simulink model "quadsim"  (R2023a)
settings: Solver=FixedStepAuto  StartTime=0.0  StopTime=tf  FixedStep=tstep  RelTol=1e-3  EnableMultiTasking=on
values from neighbouring files (symbols this model uses):
  con = [m,g,Ixx,Iyy,Izz,Ixy,Ixz,Iyz]    [main.m]
  con_real = [m_real,g_real,Ixx_real,Iyy_real,Izz_real,Ixy_real,Ixz_real,Iyz_real]    [main.m]
  KA = [-22.3606698191395	0.00201472423721912	-0.0210042926161882	-5.14256360667609	-0.00544994639254871	-0.00539750017780217	-0.591349567789534	2.56742275495149e-08	-0.000222035484653320 ... (first row only)    [main.m]
  KT = [0.0719636752505308	-0.0719636752505340	3.14585832307952	0.205167084974015	-0.205167084974022	5.80096376452051	-0.215718994756261	0.215718994756262	5.40168970403702 ... (first row only)    [main.m]
  l = 0.2    [Attitude.m]
  LA = [4.47090494564492	1.24715387948497e-08	0.00499221978617721	0.744440755445128	-4.66935645274561e-05	0.00155055930580347; 1.24715387948497e-08	4.47089657692810	5.57847618618385e-06	4.66676478608033e-05	0.744439338778690	1.57839222690215e-05; 0.00499221978617721	5.57847618618385e-06	4.46797672976086	0.000844876774321680	-2.51353961198021e-05	1.36306650125613; 0.0148888151089026	9.33352957216066e-07	1 ...(+321 chars)    [main.m]
  LT = [31.6173277650076	8.77856768873147e-05	-0.000368035074502750	1.84128362143915	3.68731318527742e-06	0.235633602584559; 8.77856768873147e-05	31.6173277650076	0.000368035074499152	3.68731318640445e-06	1.84128362143917	-0.235633602584566; -0.000368035074502750	0.000368035074499152	31.6135634683629	-0.180767234820393	0.180767234820397	2.40014416703265; 0.184128362143915	3.68731318640445e-07	-0.01807672 ...(+309 chars)    [main.m]
  ref = [pi/18 pi/32 0]    [Attitude.m]    (also in Translational.m = [0 0 -2]; main.m = [1;1;-2])
  tstep = 0.001    [ActuatorModel.m]    (also in Attitude.m; Translational.m; UpdatedAttitude.m = 0.0001; main.m)
  x0 = [0; 0; 0]    [UpdatedAttitude.m]    (also in main.m = [0;0;0;0;0;0;0;0;0;0;0;0])
undefined symbols (not defined in the file or in its folder): k1, k2, wmax
libraries: simulink x1
settings Model: Creator=Nathan Dablain  LastModifiedBy=Nathan Dablain

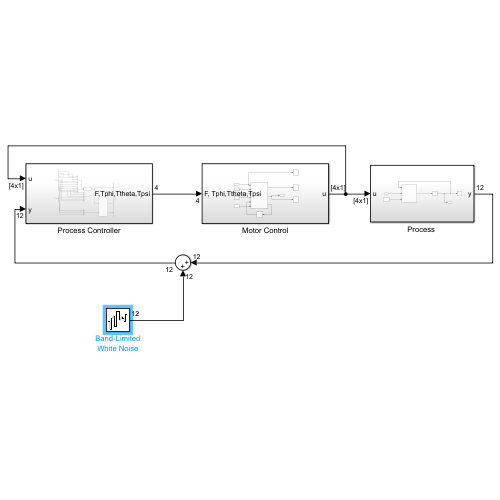
[thumbnail: Simulink's stored preview of the top-level diagram]
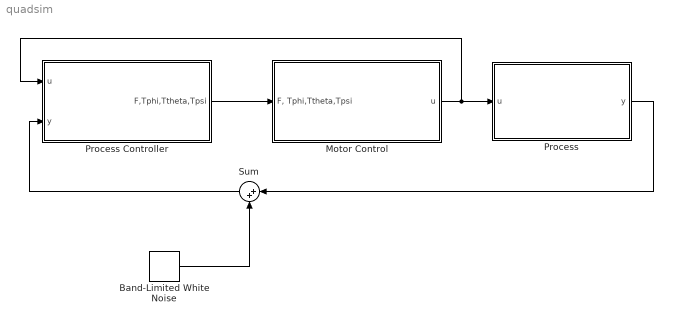
== system quadsim ==
  Band-Limited White Noise : simulink/Sources/Band-Limited White Noise  Cov=[1e-4 1e-4 1e-4 5e-5 5e-6 5e-6 1e-5 1e-5 1e-5 1e-6 1e-6 1e-6]  Ts=tstep  seed=[23341]
  Motor Control : Subsystem
  "Process " : Subsystem
  Process Controller : Subsystem
  Sum : Sum  Inputs=|++
  wires:
  Process Controller/1(F,Tphi,Ttheta,Tpsi) -> Motor Control/1("F, Tphi,Ttheta,Tpsi")
  Motor Control/1(u) -> Process Controller/1(u), "Process "/1(u)
  "Process "/1(y) -> Sum/1
  Band-Limited White Noise/1 -> Sum/2
  Sum/1 -> Process Controller/2(y)

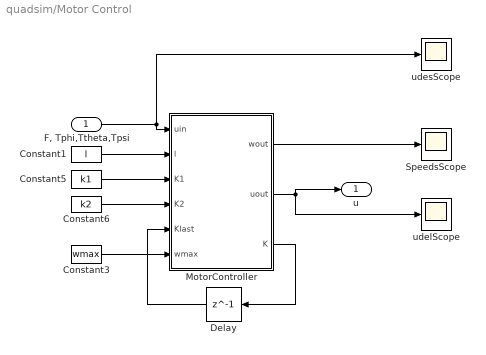
== system quadsim/Motor Control ==
  "F, Tphi,Ttheta,Tpsi" : Inport
  Constant1 : Constant  Value=l
  Constant3 : Constant  Value=wmax
  Constant5 : Constant  Value=k1
  Constant6 : Constant  Value=k2
  Delay : Delay  DelayLength=1  InitialCondition=1e-6.*ones(1,8)
  MotorController : MATLAB Function  TreatAsAtomicUnit=on
  SpeedsScope : Scope
  udelScope : Scope
  udesScope : Scope
  u : Outport
  wires:
  Constant1/1 -> MotorController/2(l)
  "F, Tphi,Ttheta,Tpsi"/1 -> udesScope/1, MotorController/1(uin)
  MotorController/2(uout) -> udelScope/1, u/1
  Constant3/1 -> MotorController/6(wmax)
  Constant5/1 -> MotorController/3(K1)
  Constant6/1 -> MotorController/4(K2)
  MotorController/1(wout) -> SpeedsScope/1
  MotorController/3(K) -> Delay/1
  Delay/1 -> MotorController/5(Klast)

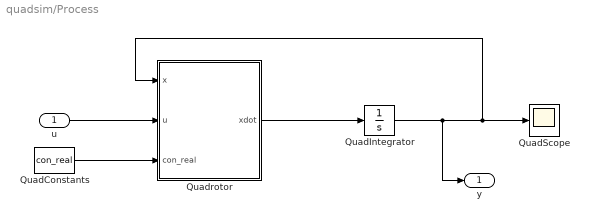
== system quadsim/Process  ==
  u : Inport
  QuadConstants : Constant  Value=con_real
  QuadIntegrator : Integrator  InitialCondition=x0
  QuadScope : Scope
  Quadrotor : MATLAB Function  TreatAsAtomicUnit=on
  y : Outport
  wires:
  u/1 -> Quadrotor/2(u)
  Quadrotor/1(xdot) -> QuadIntegrator/1
  QuadConstants/1 -> Quadrotor/3(con_real)
  QuadIntegrator/1 -> y/1, QuadScope/1, Quadrotor/1(x)

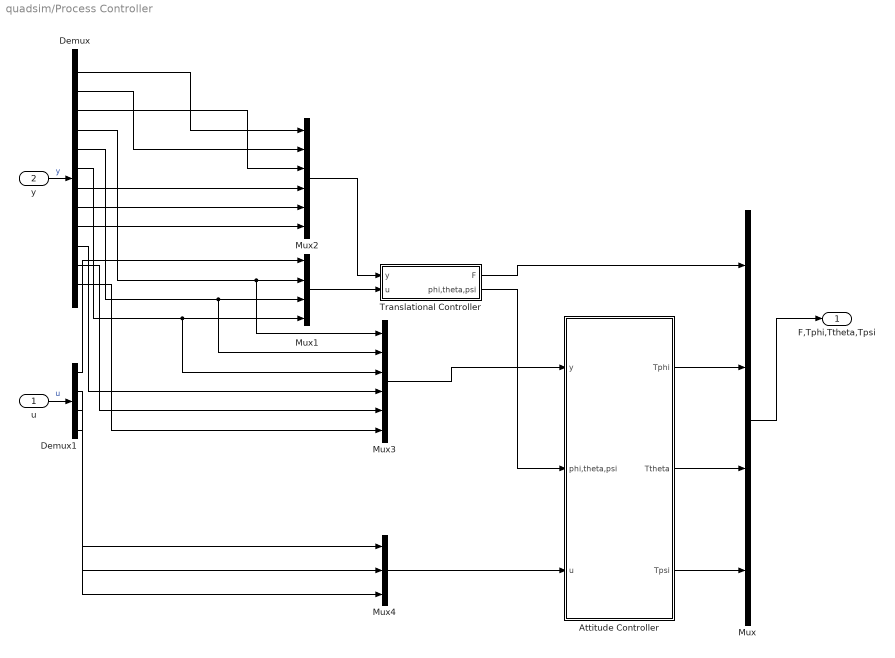
== system quadsim/Process Controller ==
  u : Inport
  y : Inport  Port=2
  Attitude Controller : Subsystem
  Demux : Demux  Outputs=12
  Demux1 : Demux
  Mux : Mux
  Mux1 : Mux
  Mux2 : Mux  Inputs=6
  Mux3 : Mux  Inputs=6
  Mux4 : Mux  Inputs=3
  Translational Controller : Subsystem
  F,Tphi,Ttheta,Tpsi : Outport
  wires:
  Mux/1 -> F,Tphi,Ttheta,Tpsi/1
  Translational Controller/1(F) -> Mux/1
  Attitude Controller/1(Tphi) -> Mux/2
  Attitude Controller/2(Ttheta) -> Mux/3
  Attitude Controller/3(Tpsi) -> Mux/4
  Translational Controller/2(phi,theta,psi) -> Attitude Controller/2(phi,theta,psi)
  Mux1/1 -> Translational Controller/2(u)
  Mux2/1 -> Translational Controller/1(y)
  Mux3/1 -> Attitude Controller/1(y)
  y/1 -> Demux/1  "y"
  u/1 -> Demux1/1  "u"
  Demux/1 -> Mux2/1
  Demux/2 -> Mux2/2
  Demux/3 -> Mux2/3
  Demux/7 -> Mux2/4
  Demux/8 -> Mux2/5
  Demux/9 -> Mux2/6
  Demux1/1 -> Mux1/1
  Demux/4 -> Mux3/1, Mux1/2
  Demux/5 -> Mux3/2, Mux1/3
  Demux/6 -> Mux3/3, Mux1/4
  Mux4/1 -> Attitude Controller/3(u)
  Demux1/2 -> Mux4/1
  Demux1/3 -> Mux4/2
  Demux1/4 -> Mux4/3
  Demux/10 -> Mux3/4
  Demux/11 -> Mux3/5
  Demux/12 -> Mux3/6

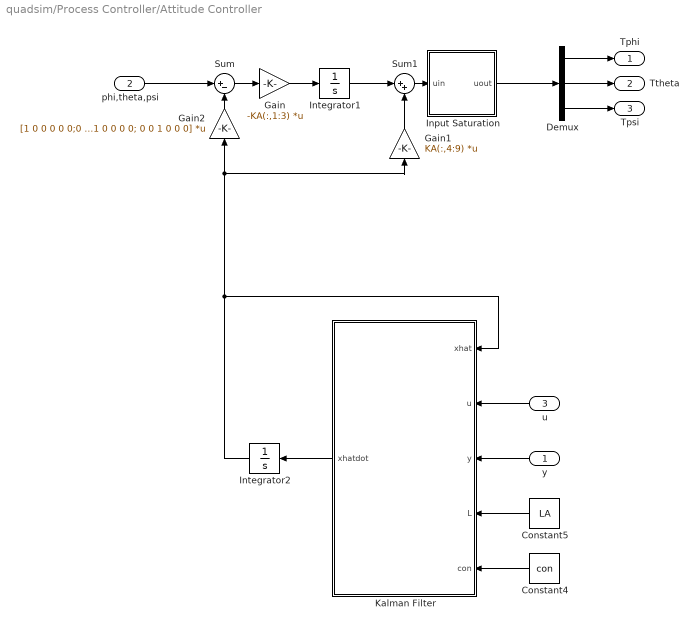
== system quadsim/Process Controller/Attitude Controller ==
  y : Inport
  phi,theta,psi : Inport  Port=2
  u : Inport  Port=3
  Constant4 : Constant  Value=con
  Constant5 : Constant  Value=LA
  Demux : Demux  Outputs=3
  Gain : Gain  Gain=-KA(:,1:3)  Multiplication=Matrix(K*u)
  Gain1 : Gain  Gain=KA(:,4:9)  Multiplication=Matrix(K*u)
  Gain2 : Gain  Gain=[1 0 0 0 0 0;0 1 0 0 0 0; 0 0 1 0 0 0]  Multiplication=Matrix(K*u)
  Input Saturation : MATLAB Function  TreatAsAtomicUnit=on
  Integrator1 : Integrator  InitialCondition=zeros(3,1)
  Integrator2 : Integrator  InitialCondition=zeros(6,1)
  Kalman Filter : MATLAB Function  TreatAsAtomicUnit=on
  Sum : Sum  Inputs=|+-
  Sum1 : Sum  Inputs=|++
  Tphi : Outport
  Ttheta : Outport  Port=2
  Tpsi : Outport  Port=3
  wires:
  phi,theta,psi/1 -> Sum/1
  Sum/1 -> Gain/1
  Gain/1 -> Integrator1/1
  Input Saturation/1(uout) -> Demux/1
  Gain1/1 -> Sum1/2
  Sum1/1 -> Input Saturation/1(uin)
  Integrator1/1 -> Sum1/1
  Demux/1 -> Tphi/1
  Demux/2 -> Ttheta/1
  Demux/3 -> Tpsi/1
  Gain2/1 -> Sum/2
  Integrator2/1 -> Kalman Filter/1(xhat), Gain1/1, Gain2/1
  Constant4/1 -> Kalman Filter/5(con)
  Kalman Filter/1(xhatdot) -> Integrator2/1
  y/1 -> Kalman Filter/3(y)
  Constant5/1 -> Kalman Filter/4(L)
  u/1 -> Kalman Filter/2(u)

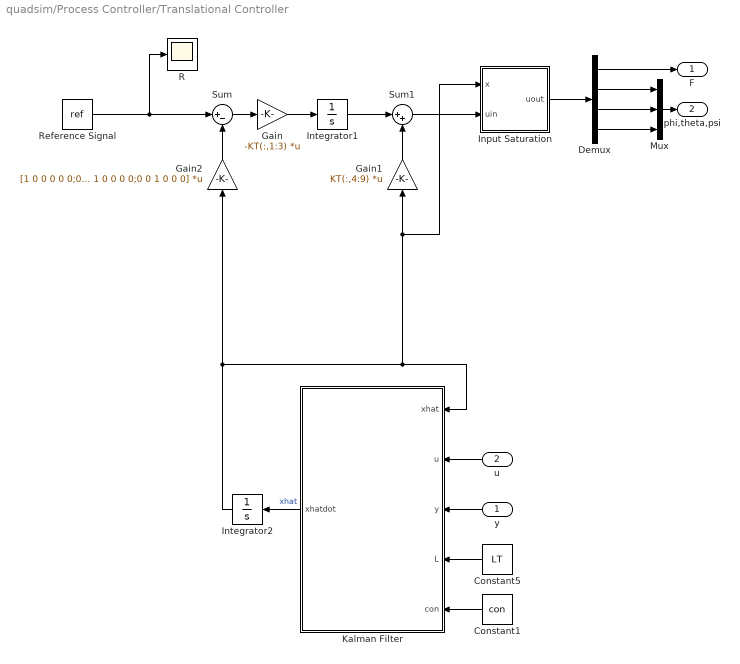
== system quadsim/Process Controller/Translational Controller ==
  y : Inport
  u : Inport  Port=2
  Constant1 : Constant  Value=con
  Constant5 : Constant  Value=LT
  Demux : Demux
  Gain : Gain  Gain=-KT(:,1:3)  Multiplication=Matrix(K*u)
  Gain1 : Gain  Gain=KT(:,4:9)  Multiplication=Matrix(K*u)
  Gain2 : Gain  Gain=[1 0 0 0 0 0;0 1 0 0 0 0;0 0 1 0 0 0]  Multiplication=Matrix(K*u)
  Input Saturation : MATLAB Function  TreatAsAtomicUnit=on
  Integrator1 : Integrator  InitialCondition=zeros(4,1)
  Integrator2 : Integrator  InitialCondition=zeros(6,1)
  Kalman Filter : MATLAB Function  TreatAsAtomicUnit=on
  Mux : Mux  Inputs=3
  R : Scope
  Reference Signal : Constant  Value=ref
  Sum : Sum  Inputs=|+-
  Sum1 : Sum  Inputs=|++
  F : Outport
  phi,theta,psi : Outport  Port=2
  wires:
  Sum1/1 -> Input Saturation/2(uin)
  Gain/1 -> Integrator1/1
  Sum/1 -> Gain/1
  Integrator1/1 -> Sum1/1
  Reference Signal/1 -> R/1, Sum/1
  Gain1/1 -> Sum1/2
  Input Saturation/1(uout) -> Demux/1
  Demux/1 -> F/1
  Demux/2 -> Mux/1
  Demux/3 -> Mux/2
  Demux/4 -> Mux/3
  Mux/1 -> phi,theta,psi/1
  Gain2/1 -> Sum/2
  Integrator2/1 -> Gain2/1, Input Saturation/1(x), Gain1/1, Kalman Filter/1(xhat)
  u/1 -> Kalman Filter/2(u)
  y/1 -> Kalman Filter/3(y)
  Constant5/1 -> Kalman Filter/4(L)
  Kalman Filter/1(xhatdot) -> Integrator2/1  "xhat"
  Constant1/1 -> Kalman Filter/5(con)

== matlab function quadsim/Process Controller/Translational Controller/Input Saturation ==
  data: x input; uin input; uout output
function uout = fcn(x,uin)
uout = uin;
max_ang = 20*pi/180; % rad
max_thrust = 30; % N
if uin(1)> max_thrust
    uout(1) = max_thrust;
elseif uin(1)<0
    uout(1) = 0;
end
for i = 2:4
    if x(3)>=-0.01
        uout(i) = 0;
    elseif uin(i) > max_ang
        uout(i) = max_ang;
    elseif uin(i) < -max_ang
        uout(i) = -max_ang;
    end
end
end

== matlab function quadsim/Process Controller/Attitude Controller/Kalman Filter ==
  data: xhat input; xhatdot output; u input; y input; L input; con input
function xhatdot  = fcn(xhat,u,y,L,con)
I = diag([con(3) con(4) con(5)]);
yhat = eye(6)*xhat;
xhatdot = [[1 sin(xhat(1))*tan(xhat(2)) cos(xhat(1))*tan(xhat(2));...
    0 cos(xhat(1)) -sin(xhat(1));...
    0 sin(xhat(1))*sec(xhat(2)) cos(xhat(1))*sec(xhat(2))]*xhat(4:6);...
    I\(u - cross(xhat(4:6),I*xhat(4:6)))] + L*(y-yhat);
end

== matlab function quadsim/Process Controller/Attitude Controller/Input Saturation ==
  data: uin input; uout output
function uout = fcn(uin)
uout = uin;
max_thrust = 30; % N
max_torque = max_thrust*0.2; % N-m
for i = 1:3
    if uin(i) > max_torque
        uout(i) = max_torque;
    elseif uin(i) < -max_torque
        uout(i) = -max_torque;
    end
end
end

== matlab function quadsim/Process Controller/Translational Controller/Kalman Filter ==
  data: xhat input; u input; y input; xhatdot output; L input; con input
function xhatdot   = fcn(xhat,u,y,L,con)
m = con(1);
g = con(2);

K = 5000; % Ground stiffness (N/m)
c = 150; % Ground damping (N/m/s)
if xhat(3) >= 0
    Fr = [c*xhat(4);c*xhat(5);K*xhat(3) + c*xhat(6)]; % Ground reaction force
else
    Fr = zeros(3,1);
end

phi = u(2);
theta = u(3);
psi = u(4);
yhat = eye(6)*xhat;
xhatdot = [[cos(theta)*cos(psi)  sin(phi)*sin(theta)*cos(psi) - cos(phi)*sin(psi) cos(phi)*sin(theta)*cos(psi)+sin(phi)*sin(psi);... 
    cos(theta)*sin(psi)  sin(phi)*sin(theta)*sin(psi)+cos(phi)*cos(psi) cos(phi)*sin(theta)*sin(psi)-sin(phi)*cos(psi);... 
    -sin(theta) sin(phi)*cos(theta) cos(phi)*cos(theta)]*xhat(4:6);...
    -g*sin(theta) - Fr(1)/m;...
    g*cos(theta)*sin(phi) - Fr(2)/m;...
    -u(1)/m-Fr(3)/m+g*cos(theta)*cos(phi)] + L*(y-yhat);
end

== matlab function quadsim/Motor Control/MotorController ==
  data: uin input; wout output; l input; K1 input; K2 input; Klast input; wmax input; uout output; K output
function [wout,uout, K] = fcn(uin, l, K1, K2, Klast, wmax)
w = zeros(4,1);
const = [Klast(1) Klast(2) Klast(3) Klast(4);...
    0 -l*Klast(2) 0 l*Klast(4);...
    -l*Klast(1) 0 l*Klast(3) 0;...
    -Klast(5) Klast(6) -Klast(7) Klast(8)];
w = const\uin;
for i = 1:4
    if w(i) <= 1
        w(i) = (2/60)^2;
    elseif sqrt(w(i))*60 >= wmax
        w(i) = (wmax/60)^2;
    end
end
K11 = K1(round(sqrt(w(1))*60)); %Because K is indexed based off of 0-7000 rpm, but n is in rps, w is rps^2
K12 = K1(round(sqrt(w(2))*60));
K13 = K1(round(sqrt(w(3))*60));
K14 = K1(round(sqrt(w(4))*60));
K21 = K2(round(sqrt(w(1))*60));
K22 = K2(round(sqrt(w(2))*60));
K23 = K2(round(sqrt(w(3))*60));
K24 = K2(round(sqrt(w(4))*60));
uout = [K11 K12 K13 K14;...
    0 -l*K12 0 l*K14;...
    -l*K11 0 l*K13 0;...
    -K21 K22 -K23 K24]*w;
wout = sqrt(w).*60; %rpm
K = [K11 K12 K13 K14 K21 K22 K23 K24]; % Pass to next loop
end

== matlab function quadsim/Process /Quadrotor ==
  data: x input; xdot output double size=12; u input; con_real input
function xdot = fcn(x,u,con_real)
%Constants: mass(1), gravity(2), Ixx(3), Iyy(4), Izz(5), Ixy(6), Ixz(7),
%Iyz(8)
I = [con_real(3) -con_real(6) -con_real(7);...
    -con_real(6) con_real(4) -con_real(8);...
    -con_real(7) -con_real(8) con_real(5)]; % MOIs and POIs
K = 500; % Ground stiffness (N/m)
C = 15; % Ground damping (N/m/s)
if x(3) > 0
    Fr = [0;0;K*x(3) + C*x(9)]; % Ground reaction force
else
    Fr = zeros(3,1);
end
M = [u(2);u(3);u(4)]; % Moments x-y-z
xdot = [[cos(x(5))*cos(x(6))  sin(x(4))*sin(x(5))*cos(x(6))-cos(x(4))*sin(x(6)) cos(x(4))*sin(x(5))*cos(x(6))+sin(x(4))*sin(x(6));... 
    cos(x(5))*sin(x(6))  sin(x(4))*sin(x(5))*sin(x(6))+cos(x(4))*cos(x(6)) cos(x(4))*sin(x(5))*sin(x(6))-sin(x(4))*cos(x(6));...
    -sin(x(5)) sin(x(4))*cos(x(5)) cos(x(4))*cos(x(5))]*x(7:9);...
    [1 sin(x(4))*tan(x(5)) cos(x(4))*tan(x(5));...
    0 cos(x(4)) -sin(x(4));...
    0 sin(x(4))*sec(x(5)) cos(x(4))*sec(x(5))]*x(10:12);...
    cross(x(7:9),x(10:12)) + con_real(2).*[-sin(x(5));cos(x(5))*sin(x(4));cos(x(5))*cos(x(4))] - [0;0;u(1)/con_real(1)] - Fr/con_real(1);...
    I\(M - cross(x(10:12),I*x(10:12)))];
end
